simulink model "controller13_AIS"  (R2020b)
settings: Solver=FixedStepDiscrete  StartTime=0.0  StopTime=inf  RelTol=1e-3
values from neighbouring files (symbols this model uses):
  ctr = make_controller()    [setup_controller_with_functions.m]
  mdl = make_model(flight_time)    [setup_controller_with_functions.m]
  ukf_P0_flat = UKF.flatten_matrix(ukf_sys.P0)    [controller_setup_ukf.m]
  ukf_prediction_time = 0.015    [controller_setup_ukf.m]
  ukf_s0 = ukf_sys.s0    [controller_setup_ukf.m]
  ukf_sys = UKF.initialize_ukf_sys(rbt, mdl, ukf_params)    [controller_setup_ukf.m]
  ukf_use_prediction = 1    [controller_setup_ukf.m]
undefined symbols (not defined in the file or in its folder): ctr1, ctr2, DiscIntNeverNeededParam, flt, IO397, rbt1, rbt2, rsim1, rsim2, som, traj2
libraries: simulink x63, slrealtimeloglib x21, slrealtimetgmanagement x8, slrealtimeseriallib x5, speedgoatlib_fpga_analog_io x4, slrealtimeutilitieslib x3, dspfdesign x2, speedgoatlib_fpga x2, slrealtimeiplib x2, speedgoatlib_fpga_dio x1
(part 2 of 5)

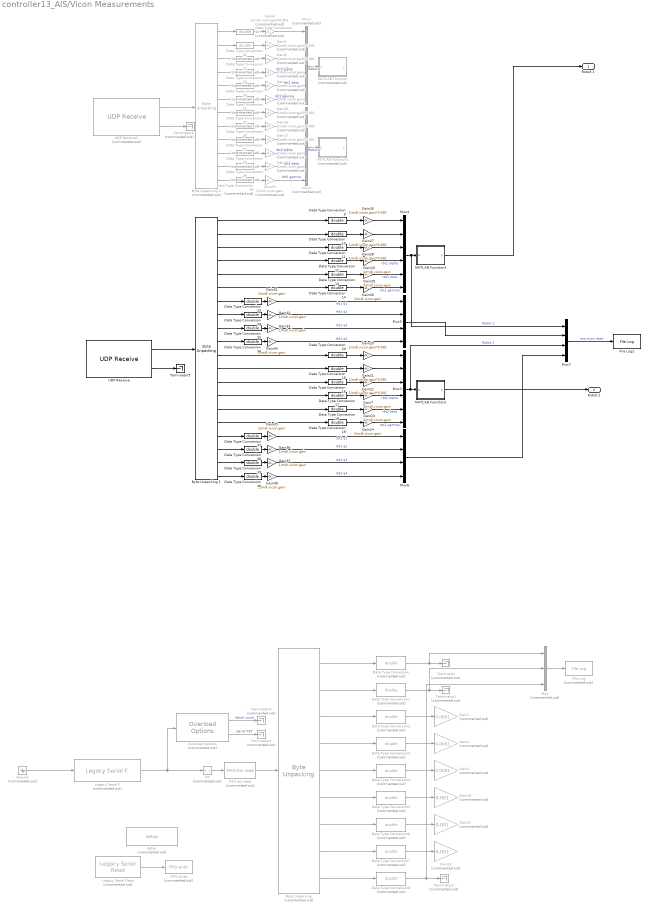
== system controller13_AIS/Vicon Measurements ==
  "Byte Unpacking " : slrealtimeutilitieslib/Byte Unpacking  Commented=on  MaskUnpackedDataTypes={'uint8','int16','int16','int16','int16','int16','int16','int16','uint8'}  MaskUnpackedDataSizes={[1] [1] [1] [1] [1] [1] [1] [1] [1]}  MaskAlignment=1
      settings: SourceProductBaseCode=XP
  Byte Unpacking 1 : slrealtimeutilitieslib/Byte Unpacking  MaskUnpackedDataTypes={'int32','int32','int32','int32','int32','int32','int32','int32','int32','int32','int32','int32','int32','int32','int32','int32','int32','int32','int32','int32'}  MaskUnpackedDataSizes={[1] [1] [1] [1] [1] [1] [1] [1] [1] [1] [1] [1] [1] [1] [1] [1] [1] [1] [1] [1]}  MaskAlignment=1
      settings: SourceProductBaseCode=XP
  Byte Unpacking 2 : slrealtimeutilitieslib/Byte Unpacking  Commented=on  MaskUnpackedDataTypes={'int32','int32','int32','int32','int32','int32','int32','int32','int32','int32','int32','int32'}  MaskUnpackedDataSizes={[1] [1] [1] [1] [1] [1] [1] [1] [1] [1] [1] [1]}  MaskAlignment=1
      settings: SourceProductBaseCode=XP
  Data Type Conversion{,1..8,21..32} (21 alike) : DataTypeConversion  Commented=on  OutDataTypeStr=double
  Data Type Conversion{9..20,33..40} (20 alike) : DataTypeConversion  OutDataTypeStr=double
  FIFO bin read : slrealtimeseriallib/FIFO bin read  Commented=on  header=[128,127,127]  lengths=[15]  hold=Hold last output if no new data  enable=off  maxsize=15  outputtype=8 bit uint null terminated  sampletime=mdl.T
      settings: SourceProductBaseCode=XP
  FIFO write : slrealtimeseriallib/FIFO write  Commented=on  size=1024  inputtype=count+16 bit uint  present=off  sampletime=-1
      settings: SourceProductBaseCode=XP
  File Log : slrealtimeloglib/File Log  Commented=on  decimation=1
      settings: SourceProductBaseCode=XP
  File Log1 : slrealtimeloglib/File Log  decimation=1
      settings: SourceProductBaseCode=XP
  Gain1 : Gain  Commented=on  Gain=0.0001
  Gain10 : Gain  Commented=on  Gain=0.001
  Gain11 : Gain  Commented=on  Gain=0.001
  Gain12 : Gain  Commented=on  Gain=0.001
  Gain{8..9,13..14,18..19} (6 alike) : Gain  Commented=on  Gain=1/mdl.vicon.gain
  Gain{4..6,15..17} (6 alike) : Gain  Commented=on  Gain=1/mdl.vicon.gain*0.001
  Gain2 : Gain  Commented=on  Gain=0.0001
  Gain{20..22,26..28} (6 alike) : Gain  Gain=1/mdl.vicon.gain*0.001
  Gain{7,23..25,29..38} (14 alike) : Gain  Gain=1/mdl.vicon.gain
  Gain3 : Gain  Commented=on  Gain=0.0001
  Ground : Ground  Commented=on
  Legacy Serial F : slrealtimeseriallib/Mainboard/Legacy Serial F  Commented=on  port=Legacy Serial Port 1  baud=115200  width=8  nstop=1  parity=None  ctsmode=on  idtype=8 bit uint null terminated  sampletime=0.0005
      settings: SourceProductBaseCode=XP
  Legacy Serial Read : slrealtimeseriallib/Mainboard/Legacy Serial Read  Commented=on  port=Legacy Serial Port 1  count=51  dtype=count+16 bit uint  sampletime=mdl.T
      settings: SourceProductBaseCode=XP
  MATLAB Function : MATLAB Function  Commented=on  TreatAsAtomicUnit=on  SystemSampleTime=mdl.T
  MATLAB Function1 : MATLAB Function  Commented=on  TreatAsAtomicUnit=on  SystemSampleTime=mdl.T
  MATLAB Function2 : MATLAB Function  TreatAsAtomicUnit=on  SystemSampleTime=mdl.T
  MATLAB Function3 : MATLAB Function  TreatAsAtomicUnit=on  SystemSampleTime=mdl.T
  Mux : Mux  Commented=on  Inputs=3
  Mux1 : Mux  Commented=on  Inputs=6
  Mux2 : Mux  Commented=on  Inputs=6
  Mux3 : Mux  Inputs=6
  Mux4 : Mux  Inputs=6
  Mux5 : Mux
  Mux6 : Mux
  Mux7 : Mux
  Overload Options : slrealtimetgmanagement/Overload Options  Commented=on  startupDur=10  startupDurSrc=Tunable Parameter  maxOverload=10  maxOverloadSrc=Tunable Parameter  TETFlag=on
      settings: SourceProductBaseCode=XP
  RT : RateTransition  Commented=on  Integrity=off  OutPortSampleTime=mdl.T
  Setup : slrealtimeseriallib/Mainboard/Setup  Commented=on  port=Legacy Serial Port 1  baud=115200  width=8  nstop=1  parity=None  ctsmode=on
      settings: SourceProductBaseCode=XP
  Terminator{,1..4,6} (6 alike) : Terminator  Commented=on
  Terminator5 : Terminator
  UDP Receive : slrealtimeiplib/UDP Receive  useHostTargetConn=off  ipAddress=192.168.8.11  localPort=1024  rcvWidth=80  rcvFmAny=on  fmAddress=192.168.7.11  rcvMulticast=off  multicastAddress={}  sampleTime=1/2500
      settings: SourceProductBaseCode=XP
  UDP Receive1 : slrealtimeiplib/UDP Receive  Commented=on  useHostTargetConn=off  ipAddress=192.168.8.11  localPort=1024  rcvWidth=48  rcvFmAny=on  fmAddress=192.168.7.11  rcvMulticast=off  multicastAddress={}  sampleTime=1/2500
      settings: SourceProductBaseCode=XP
  Robot 1 : Outport
  Robot 2 : Outport  Port=2
  wires:
  "Byte Unpacking "/3 -> Data Type Conversion2/1
  Data Type Conversion2/1 -> Gain1/1
  "Byte Unpacking "/9 -> Data Type Conversion8/1
  "Byte Unpacking "/4 -> Data Type Conversion3/1
  Data Type Conversion6/1 -> Gain11/1
  Data Type Conversion4/1 -> Gain3/1
  "Byte Unpacking "/2 -> Data Type Conversion1/1
  Data Type Conversion5/1 -> Gain10/1
  Data Type Conversion7/1 -> Gain12/1
  "Byte Unpacking "/6 -> Data Type Conversion5/1
  "Byte Unpacking "/8 -> Data Type Conversion7/1
  Data Type Conversion3/1 -> Gain2/1
  "Byte Unpacking "/5 -> Data Type Conversion4/1
  "Byte Unpacking "/7 -> Data Type Conversion6/1
  "Byte Unpacking "/1 -> Data Type Conversion/1
  Legacy Serial Read/1 -> FIFO write/1
  FIFO bin read/1 -> "Byte Unpacking "/1
  Ground/1 -> Legacy Serial F/1
  Legacy Serial F/1 -> Overload Options/1, RT/1
  RT/1 -> FIFO bin read/1
  Data Type Conversion/1 -> Mux/1, Terminator/1
  Data Type Conversion1/1 -> Mux/2, Terminator1/1
  Data Type Conversion8/1 -> Mux/3, Terminator2/1
  Mux/1 -> File Log/1
  Overload Options/1 -> Terminator4/1  "Serial count"
  Overload Options/2 -> Terminator3/1  "Serial TET"
  UDP Receive/2 -> Terminator5/1
  UDP Receive/1 -> Byte Unpacking 1/1
  Byte Unpacking 1/1 -> Data Type Conversion9/1
  Byte Unpacking 1/2 -> Data Type Conversion10/1
  Byte Unpacking 1/3 -> Data Type Conversion11/1
  Byte Unpacking 1/4 -> Data Type Conversion12/1
  Byte Unpacking 1/5 -> Data Type Conversion13/1
  Byte Unpacking 1/6 -> Data Type Conversion14/1
  Gain4/1 -> Mux1/1
  Gain5/1 -> Mux1/2
  Gain6/1 -> Mux1/3
  Gain13/1 -> Mux1/4  "rbt1 alpha"
  Gain8/1 -> Mux1/5  "rbt1 beta"
  Gain9/1 -> Mux1/6  "rbt1 gamma"
  Gain15/1 -> Mux2/1
  Gain16/1 -> Mux2/2
  Gain17/1 -> Mux2/3
  Gain14/1 -> Mux2/4  "rbt2 alpha"
  Gain18/1 -> Mux2/5  "rbt2 beta"
  Gain19/1 -> Mux2/6  "rbt2 gamma"
  Mux1/1 -> MATLAB Function/1(u)  "Robot 1"
  Mux2/1 -> MATLAB Function1/1(u)  "Robot 2"
  Byte Unpacking 2/12 -> Data Type Conversion30/1
  Byte Unpacking 2/9 -> Data Type Conversion27/1
  Byte Unpacking 2/7 -> Data Type Conversion31/1
  Byte Unpacking 2/3 -> Data Type Conversion22/1
  Byte Unpacking 2/6 -> Data Type Conversion25/1
  Byte Unpacking 2/4 -> Data Type Conversion23/1
  Byte Unpacking 2/10 -> Data Type Conversion28/1
  UDP Receive1/2 -> Terminator6/1
  Byte Unpacking 2/2 -> Data Type Conversion21/1
  Byte Unpacking 2/8 -> Data Type Conversion26/1
  UDP Receive1/1 -> Byte Unpacking 2/1
  Byte Unpacking 2/1 -> Data Type Conversion32/1
  Byte Unpacking 2/11 -> Data Type Conversion29/1
  Byte Unpacking 2/5 -> Data Type Conversion24/1
  Byte Unpacking 1/11 -> Data Type Conversion20/1
  Byte Unpacking 1/12 -> Data Type Conversion15/1
  Byte Unpacking 1/13 -> Data Type Conversion16/1
  Byte Unpacking 1/14 -> Data Type Conversion17/1
  Byte Unpacking 1/15 -> Data Type Conversion18/1
  Byte Unpacking 1/16 -> Data Type Conversion19/1
  Data Type Conversion33/1 -> Gain31/1
  Gain31/1 -> Mux5/1  "rbt1 q1"
  Byte Unpacking 1/7 -> Data Type Conversion33/1
  Data Type Conversion34/1 -> Gain32/1
  Gain32/1 -> Mux5/2  "rbt1 q2"
  Byte Unpacking 1/8 -> Data Type Conversion34/1
  Data Type Conversion35/1 -> Gain33/1
  Data Type Conversion36/1 -> Gain34/1
  Byte Unpacking 1/9 -> Data Type Conversion35/1
  Byte Unpacking 1/10 -> Data Type Conversion36/1
  Gain33/1 -> Mux5/3  "rbt1 q3"
  Gain34/1 -> Mux5/4  "rbt1 q4"
  Gain38/1 -> Mux6/4  "rbt2 q4"
  Gain37/1 -> Mux6/3  "rbt2 q3"
  Data Type Conversion37/1 -> Gain35/1
  Gain35/1 -> Mux6/1  "rbt2 q1"
  Data Type Conversion40/1 -> Gain38/1
  Data Type Conversion38/1 -> Gain36/1
  Gain36/1 -> Mux6/2  "rbt2 q2"
  Data Type Conversion39/1 -> Gain37/1
  Byte Unpacking 1/17 -> Data Type Conversion37/1
  Byte Unpacking 1/18 -> Data Type Conversion38/1
  Byte Unpacking 1/19 -> Data Type Conversion39/1
  Byte Unpacking 1/20 -> Data Type Conversion40/1
  Data Type Conversion32/1 -> Gain4/1
  Data Type Conversion21/1 -> Gain5/1
  Data Type Conversion23/1 -> Gain13/1
  Data Type Conversion22/1 -> Gain6/1
  Data Type Conversion24/1 -> Gain8/1
  Data Type Conversion25/1 -> Gain9/1
  Data Type Conversion31/1 -> Gain15/1
  Data Type Conversion26/1 -> Gain16/1
  Data Type Conversion27/1 -> Gain17/1
  Data Type Conversion28/1 -> Gain14/1
  Data Type Conversion29/1 -> Gain18/1
  Data Type Conversion30/1 -> Gain19/1
  Gain23/1 -> Mux3/5  "rbt2 beta"
  Gain7/1 -> Mux3/4  "rbt2 alpha"
  Gain22/1 -> Mux3/3
  Mux3/1 -> Mux7/3, MATLAB Function2/1(u)  "Robot 2"
  Gain24/1 -> Mux3/6  "rbt2 gamma"
  Gain20/1 -> Mux3/1
  Gain21/1 -> Mux3/2
  Data Type Conversion20/1 -> Gain20/1
  Data Type Conversion15/1 -> Gain21/1
  Data Type Conversion16/1 -> Gain22/1
  Data Type Conversion17/1 -> Gain7/1
  Data Type Conversion18/1 -> Gain23/1
  Data Type Conversion19/1 -> Gain24/1
  Gain26/1 -> Mux4/1
  Gain27/1 -> Mux4/2
  Gain30/1 -> Mux4/6  "rbt1 gamma"
  Mux4/1 -> Mux7/1, MATLAB Function3/1(u)  "Robot 1"
  Gain28/1 -> Mux4/3
  Gain29/1 -> Mux4/5  "rbt1 beta"
  Gain25/1 -> Mux4/4  "rbt1 alpha"
  Data Type Conversion9/1 -> Gain26/1
  Data Type Conversion10/1 -> Gain27/1
  Data Type Conversion11/1 -> Gain28/1
  Data Type Conversion12/1 -> Gain25/1
  Data Type Conversion13/1 -> Gain29/1
  Data Type Conversion14/1 -> Gain30/1
  MATLAB Function3/1(y) -> Robot 1/1
  MATLAB Function2/1(y) -> Robot 2/1
  Mux7/1 -> File Log1/1  "raw vicon data"
  Mux5/1 -> Mux7/2
  Mux6/1 -> Mux7/4

== system controller13_AIS/closed loop en 1 ==
  x tor : Inport
  y tor : Inport  Port=2
  z tor : Inport  Port=3
  thurst : Inport  Port=4
  enable : Constant  Value=ctr1.en
  enable{1..4} (4 alike) : Product  Inputs=**
  safety1 : Subsystem
  safety2 : Subsystem
  safety3 : Subsystem
  safety4 : Subsystem
  tor x : Outport
  tor y : Outport  Port=2
  tor z : Outport  Port=3
  Force : Outport  Port=4
  wires:
  enable/1 -> enable2/1, enable3/1, enable4/1, enable1/1
  z tor/1 -> enable3/2
  y tor/1 -> enable2/2
  x tor/1 -> enable1/2
  thurst/1 -> enable4/2
  enable1/1 -> safety1/1(In1)
  enable2/1 -> safety2/1(In1)
  enable3/1 -> safety3/1(In1)
  enable4/1 -> safety4/1(In1)
  safety1/1(Out1) -> tor x/1
  safety2/1(Out1) -> tor y/1
  safety3/1(Out1) -> tor z/1
  safety4/1(Out1) -> Force/1

== system controller13_AIS/closed loop en 2 ==
  x tor : Inport
  y tor : Inport  Port=2
  z tor : Inport  Port=3
  thurst : Inport  Port=4
  enable : Constant  Value=ctr2.en
  enable{1..4} (4 alike) : Product  Inputs=**
  safety1 : Subsystem
  safety2 : Subsystem
  safety3 : Subsystem
  safety4 : Subsystem
  tor x : Outport
  tor y : Outport  Port=2
  tor z : Outport  Port=3
  Force : Outport  Port=4
  wires:
  enable/1 -> enable2/1, enable3/1, enable4/1, enable1/1
  z tor/1 -> enable3/2
  y tor/1 -> enable2/2
  x tor/1 -> enable1/2
  thurst/1 -> enable4/2
  enable1/1 -> safety1/1(In1)
  enable2/1 -> safety2/1(In1)
  enable3/1 -> safety3/1(In1)
  enable4/1 -> safety4/1(In1)
  safety1/1(Out1) -> tor x/1
  safety2/1(Out1) -> tor y/1
  safety3/1(Out1) -> tor z/1
  safety4/1(Out1) -> Force/1

== system controller13_AIS/counter 1 ==
  running time : Inport
  Add : Sum  Inputs=+-
  Add1 : Sum
  Compare To Zero : simulink/Logic and Bit Operations/Compare To Zero  relop=<  OutDataTypeStr=uint8  ZeroCross=off
  Product2 : Product  RndMeth=Zero
  Relational Operator : RelationalOperator  Operator=>  OutDataTypeStr=boolean  RndMeth=Simplest
  SaturatingRamp : DiscreteIntegrator  gainval=1  SampleTime=-1  UpperSaturationLimit=1  LowerSaturationLimit=0  ICPrevOutput=DiscIntNeverNeededParam  ICPrevScaledInput=DiscIntNeverNeededParam
  Stop Simulation : Stop
  constant : Constant
  start delay compare : simulink/Logic and Bit Operations/Compare To Constant  relop=>  const=mdl.i_delay  OutDataTypeStr=uint8
  enable : Outport
  wires:
  SaturatingRamp/1 -> Relational Operator/1, Add/1, start delay compare/1
  running time/1 -> Add1/2, Add/2
  Add/1 -> Compare To Zero/1
  start delay compare/1 -> Product2/1
  Compare To Zero/1 -> Product2/2
  Product2/1 -> enable/1
  constant/1 -> Add1/1, SaturatingRamp/1
  Relational Operator/1 -> Stop Simulation/1
  Add1/1 -> Relational Operator/2

== system controller13_AIS/counter 2 ==
  running time : Inport
  Add : Sum  Inputs=+-
  Add1 : Sum
  Compare To Zero : simulink/Logic and Bit Operations/Compare To Zero  relop=<  OutDataTypeStr=uint8  ZeroCross=off
  Product2 : Product  RndMeth=Zero
  Relational Operator : RelationalOperator  Operator=>  OutDataTypeStr=boolean  RndMeth=Simplest
  SaturatingRamp : DiscreteIntegrator  gainval=1  SampleTime=-1  UpperSaturationLimit=1  LowerSaturationLimit=0  ICPrevOutput=DiscIntNeverNeededParam  ICPrevScaledInput=DiscIntNeverNeededParam
  Stop Simulation : Stop
  constant : Constant
  start delay compare : simulink/Logic and Bit Operations/Compare To Constant  relop=>  const=mdl.i_delay  OutDataTypeStr=uint8
  enable : Outport
  wires:
  SaturatingRamp/1 -> Relational Operator/1, Add/1, start delay compare/1
  running time/1 -> Add1/2, Add/2
  Add/1 -> Compare To Zero/1
  start delay compare/1 -> Product2/1
  Compare To Zero/1 -> Product2/2
  Product2/1 -> enable/1
  constant/1 -> Add1/1, SaturatingRamp/1
  Relational Operator/1 -> Stop Simulation/1
  Add1/1 -> Relational Operator/2

== system controller13_AIS/disturbance 1 ==
  Constant : Constant  Value=rsim1.dist.pos.en
  Constant1 : Constant  Value=[0;0;0;]
  Constant2 : Constant  Value=rsim1.dist.rot.en
  Constant3 : Constant  Value=[0;0;0;]
  Mux1 : Mux  Inputs=3
  Mux2 : Mux  Inputs=3
  Mux3 : Mux  Inputs=2
  Random Number : RandomNumber  Mean=rsim1.dist.x.mean  Variance=rsim1.dist.x.var  Seed=rsim1.dist.x.seed
  Random Number1 : RandomNumber  Mean=rsim1.dist.y.mean  Variance=rsim1.dist.y.var  Seed=rsim1.dist.y.seed
  Random Number2 : RandomNumber  Mean=rsim1.dist.z.mean  Variance=rsim1.dist.z.var  Seed=rsim1.dist.z.seed
  Random Number3 : RandomNumber  Mean=rsim1.dist.wx.mean  Variance=rsim1.dist.wx.var  Seed=rsim1.dist.wx.seed
  Random Number4 : RandomNumber  Mean=rsim1.dist.wy.mean  Variance=rsim1.dist.wy.var  Seed=rsim1.dist.wy.seed
  Random Number5 : RandomNumber  Mean=rsim1.dist.wz.mean  Variance=rsim1.dist.wz.var  Seed=rsim1.dist.wz.seed
  Switch : Switch  Threshold=1
  Switch1 : Switch  Threshold=1
  disturbance : Outport  VectorParamsAs1DForOutWhenUnconnected=off
  wires:
  Random Number/1 -> Mux1/1
  Random Number2/1 -> Mux1/3
  Mux1/1 -> Switch/1
  Random Number1/1 -> Mux1/2
  Switch/1 -> Mux3/1
  Constant/1 -> Switch/2
  Constant1/1 -> Switch/3
  Mux2/1 -> Switch1/1
  Random Number5/1 -> Mux2/3
  Constant3/1 -> Switch1/3
  Constant2/1 -> Switch1/2
  Random Number4/1 -> Mux2/2
  Random Number3/1 -> Mux2/1
  Switch1/1 -> Mux3/2
  Mux3/1 -> disturbance/1

== system controller13_AIS/disturbance 2 ==
  Constant : Constant  Value=rsim2.dist.pos.en
  Constant1 : Constant  Value=[0;0;0;]
  Constant2 : Constant  Value=rsim2.dist.rot.en
  Constant3 : Constant  Value=[0;0;0;]
  Mux1 : Mux  Inputs=3
  Mux2 : Mux  Inputs=3
  Mux3 : Mux  Inputs=2
  Random Number : RandomNumber  Mean=rsim2.dist.x.mean  Variance=rsim2.dist.x.var  Seed=rsim2.dist.x.seed
  Random Number1 : RandomNumber  Mean=rsim2.dist.y.mean  Variance=rsim2.dist.y.var  Seed=rsim2.dist.y.seed
  Random Number2 : RandomNumber  Mean=rsim2.dist.z.mean  Variance=rsim2.dist.z.var  Seed=rsim2.dist.z.seed
  Random Number3 : RandomNumber  Mean=rsim2.dist.wx.mean  Variance=rsim2.dist.wx.var  Seed=rsim2.dist.wx.seed
  Random Number4 : RandomNumber  Mean=rsim2.dist.wy.mean  Variance=rsim2.dist.wy.var  Seed=rsim2.dist.wy.seed
  Random Number5 : RandomNumber  Mean=rsim2.dist.wz.mean  Variance=rsim2.dist.wz.var  Seed=rsim2.dist.wz.seed
  Switch : Switch  Threshold=1
  Switch1 : Switch  Threshold=1
  disturbance : Outport  VectorParamsAs1DForOutWhenUnconnected=off
  wires:
  Random Number/1 -> Mux1/1
  Random Number2/1 -> Mux1/3
  Mux1/1 -> Switch/1
  Random Number1/1 -> Mux1/2
  Switch/1 -> Mux3/1
  Constant/1 -> Switch/2
  Constant1/1 -> Switch/3
  Mux2/1 -> Switch1/1
  Random Number5/1 -> Mux2/3
  Constant3/1 -> Switch1/3
  Constant2/1 -> Switch1/2
  Random Number4/1 -> Mux2/2
  Random Number3/1 -> Mux2/1
  Switch1/1 -> Mux3/2
  Mux3/1 -> disturbance/1

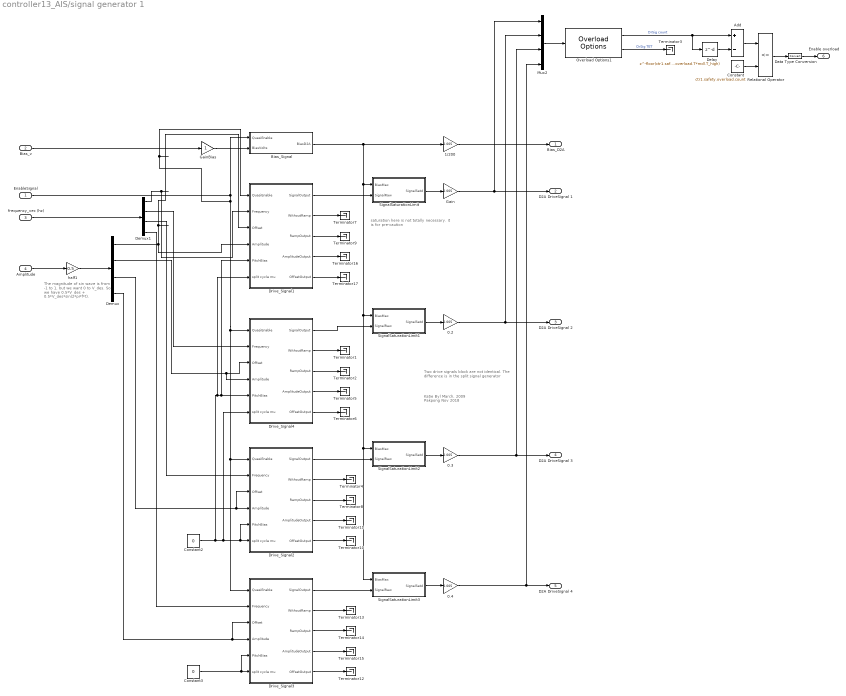
== system controller13_AIS/signal generator 1 ==
  note: The magnitude of sin wave is from -1 to 1, but we want 0 to V_des. So we have 0.5*V_des + 0.5*V_des*sin(2*pi*f*t).
  note: Katie Byl
      | March, 2009
      |
      | Pakpong
      | Nov 2018
  note: Two drive signals block are not identical.
      | The difference is in the split signal generator
  note: saturation here is not totally necessary.
      | it is for pre-caution
  EnableSignal : Inport
  Bias_v : Inport  Port=2
  frequency_vec (hz) : Inport  Port=3
  Amplitude : Inport  Port=4
  0.2 : Gain  Gain=0.005
  0.3 : Gain  Gain=0.005
  0.4 : Gain  Gain=0.005
  1/200 : Gain  Gain=0.005
  Add : Sum  Inputs=+-
  Bias_Signal : Subsystem
  Constant : Constant  Value=ctr1.safety.overload.count
  Constant2 : Constant  Value=0
  Constant3 : Constant  Value=0
  Data Type Conversion : DataTypeConversion
  Delay : Delay  DelayLength=floor(ctr1.safety.overload.T*mdl.T_high)  InitialCondition=0
  Demux : Demux
  Demux1 : Demux
  Drive_Signal1 : Subsystem
  Drive_Signal2 : Subsystem
  Drive_Signal3 : Subsystem
  Drive_Signal4 : Subsystem
  Gain : Gain  Gain=0.005
  GainBias : Gain
  Mux2 : Mux
  Overload Options1 : slrealtimetgmanagement/Overload Options  startupDur=10  startupDurSrc=Tunable Parameter  maxOverload=1000  maxOverloadSrc=Tunable Parameter  TETFlag=on
      settings: SourceProductBaseCode=XP
  Relational Operator : RelationalOperator  Operator=<=  OutDataTypeStr=boolean  RndMeth=Simplest
  SignalSaturationLimit : Subsystem
  SignalSaturationLimit1 : Subsystem
  SignalSaturationLimit2 : Subsystem
  SignalSaturationLimit3 : Subsystem
  Terminator{1..17} (17 alike) : Terminator
  half1 : Gain  Gain=0.5
  Bias_D2A : Outport
  D2A DriveSignal 1 : Outport  Port=2
  D2A DriveSignal 2 : Outport  Port=3
  D2A DriveSignal 3 : Outport  Port=4
  D2A DriveSignal 4 : Outport  Port=5
  Enable overload : Outport  Port=6
  wires:
  Bias_Signal/1(BiasD2A) -> SignalSaturationLimit3/1(BiasMax), SignalSaturationLimit2/1(BiasMax), SignalSaturationLimit1/1(BiasMax), SignalSaturationLimit/1(BiasMax), 1/200/1
  Bias_v/1 -> GainBias/1
  EnableSignal/1 -> Drive_Signal1/1(QuasiEnable), Drive_Signal3/1(QuasiEnable), Drive_Signal2/1(QuasiEnable), Drive_Signal4/1(QuasiEnable), Bias_Signal/1(QuasiEnable)
  SignalSaturationLimit/1(SignalSatd) -> Gain/1
  GainBias/1 -> Bias_Signal/2(BiasVolts)
  SignalSaturationLimit1/1(SignalSatd) -> 0.2/1
  Amplitude/1 -> half1/1
  1/200/1 -> Bias_D2A/1
  Gain/1 -> Mux2/1, D2A DriveSignal 1/1
  Drive_Signal3/4(AmplitudeOutput) -> Terminator15/1
  Drive_Signal3/2(WithoutRamp) -> Terminator13/1
  Drive_Signal3/3(RampOutput) -> Terminator14/1
  Drive_Signal3/5(OffsetOutput) -> Terminator12/1
  Drive_Signal2/3(RampOutput) -> Terminator8/1
  Drive_Signal2/4(AmplitudeOutput) -> Terminator11/1
  Drive_Signal3/1(SignalOutput) -> SignalSaturationLimit3/2(SignalRaw)
  Drive_Signal2/5(OffsetOutput) -> Terminator10/1
  Drive_Signal2/2(WithoutRamp) -> Terminator4/1
  Demux/2 -> Drive_Signal4/4(Amplitude), Drive_Signal4/3(Offset)
  Demux/3 -> Drive_Signal2/4(Amplitude), Drive_Signal2/3(Offset)
  Demux/4 -> Drive_Signal3/4(Amplitude), Drive_Signal3/3(Offset)
  Constant2/1 -> Drive_Signal1/6(split cycle mu), Drive_Signal1/5(PitchBias), Drive_Signal4/5(PitchBias), Drive_Signal4/6(split cycle mu), Drive_Signal2/5(PitchBias), Drive_Signal2/6(split cycle mu)
  Constant3/1 -> Drive_Signal3/5(PitchBias), Drive_Signal3/6(split cycle mu)
  0.3/1 -> D2A DriveSignal 3/1, Mux2/3
  SignalSaturationLimit2/1(SignalSatd) -> 0.3/1
  0.4/1 -> D2A DriveSignal 4/1, Mux2/4
  SignalSaturationLimit3/1(SignalSatd) -> 0.4/1
  Drive_Signal2/1(SignalOutput) -> SignalSaturationLimit2/2(SignalRaw)
  half1/1 -> Demux/1
  frequency_vec (hz)/1 -> Demux1/1
  Demux1/1 -> Drive_Signal1/2(Frequency)
  Demux1/2 -> Drive_Signal4/2(Frequency)
  Demux1/3 -> Drive_Signal2/2(Frequency)
  Demux1/4 -> Drive_Signal3/2(Frequency)
  0.2/1 -> Mux2/2, D2A DriveSignal 2/1
  Overload Options1/1 -> Delay/1, Add/1  "DrSig count"
  Overload Options1/2 -> Terminator3/1  "DrSig TET"
  Mux2/1 -> Overload Options1/1
  Delay/1 -> Add/2
  Add/1 -> Relational Operator/1
  Constant/1 -> Relational Operator/2
  Relational Operator/1 -> Data Type Conversion/1
  Data Type Conversion/1 -> Enable overload/1
  Drive_Signal4/1(SignalOutput) -> SignalSaturationLimit1/2(SignalRaw)
  Drive_Signal4/2(WithoutRamp) -> Terminator1/1
  Drive_Signal4/3(RampOutput) -> Terminator2/1
  Drive_Signal4/4(AmplitudeOutput) -> Terminator5/1
  Drive_Signal4/5(OffsetOutput) -> Terminator6/1
  Drive_Signal1/4(AmplitudeOutput) -> Terminator16/1
  Drive_Signal1/1(SignalOutput) -> SignalSaturationLimit/2(SignalRaw)
  Drive_Signal1/2(WithoutRamp) -> Terminator7/1
  Drive_Signal1/5(OffsetOutput) -> Terminator17/1
  Drive_Signal1/3(RampOutput) -> Terminator9/1
  Demux/1 -> Drive_Signal1/3(Offset), Drive_Signal1/4(Amplitude)

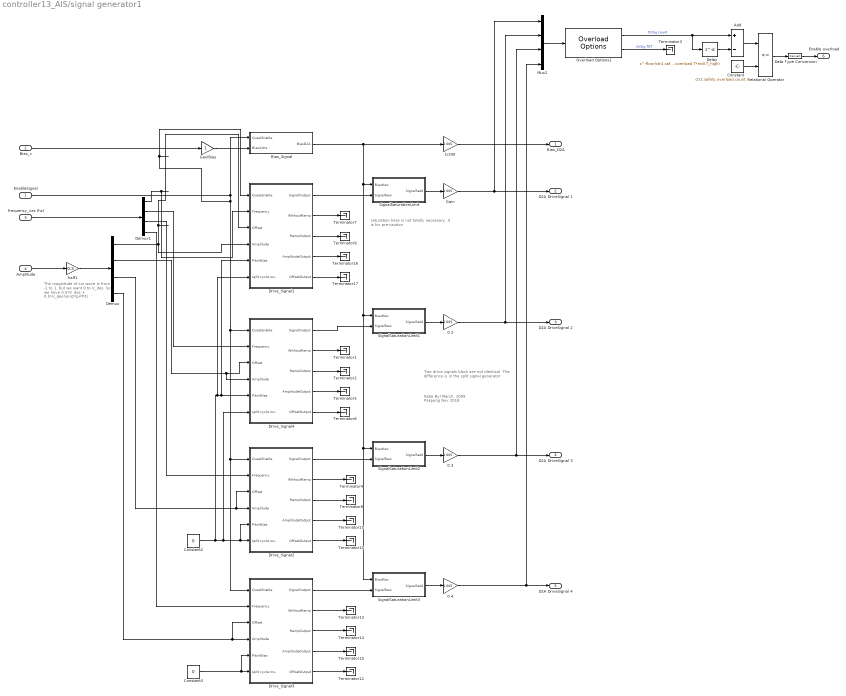
== system controller13_AIS/signal generator1 ==
  note: The magnitude of sin wave is from -1 to 1, but we want 0 to V_des. So we have 0.5*V_des + 0.5*V_des*sin(2*pi*f*t).
  note: Katie Byl
      | March, 2009
      |
      | Pakpong
      | Nov 2018
  note: Two drive signals block are not identical.
      | The difference is in the split signal generator
  note: saturation here is not totally necessary.
      | it is for pre-caution
  EnableSignal : Inport
  Bias_v : Inport  Port=2
  frequency_vec (hz) : Inport  Port=3
  Amplitude : Inport  Port=4
  0.2 : Gain  Gain=0.005
  0.3 : Gain  Gain=0.005
  0.4 : Gain  Gain=0.005
  1/200 : Gain  Gain=0.005
  Add : Sum  Inputs=+-
  Bias_Signal : Subsystem
  Constant : Constant  Value=ctr2.safety.overload.count
  Constant2 : Constant  Value=0
  Constant3 : Constant  Value=0
  Data Type Conversion : DataTypeConversion
  Delay : Delay  DelayLength=floor(ctr2.safety.overload.T*mdl.T_high)  InitialCondition=0
  Demux : Demux
  Demux1 : Demux
  Drive_Signal1 : Subsystem
  Drive_Signal2 : Subsystem
  Drive_Signal3 : Subsystem
  Drive_Signal4 : Subsystem
  Gain : Gain  Gain=0.005
  GainBias : Gain
  Mux2 : Mux
  Overload Options1 : slrealtimetgmanagement/Overload Options  startupDur=10  startupDurSrc=Tunable Parameter  maxOverload=1000  maxOverloadSrc=Tunable Parameter  TETFlag=on
      settings: SourceProductBaseCode=XP
  Relational Operator : RelationalOperator  Operator=<=  OutDataTypeStr=boolean  RndMeth=Simplest
  SignalSaturationLimit : Subsystem
  SignalSaturationLimit1 : Subsystem
  SignalSaturationLimit2 : Subsystem
  SignalSaturationLimit3 : Subsystem
  Terminator{1..17} (17 alike) : Terminator
  half1 : Gain  Gain=0.5
  Bias_D2A : Outport
  D2A DriveSignal 1 : Outport  Port=2
  D2A DriveSignal 2 : Outport  Port=3
  D2A DriveSignal 3 : Outport  Port=4
  D2A DriveSignal 4 : Outport  Port=5
  Enable overload : Outport  Port=6
  wires:
  Bias_Signal/1(BiasD2A) -> SignalSaturationLimit3/1(BiasMax), SignalSaturationLimit2/1(BiasMax), SignalSaturationLimit1/1(BiasMax), SignalSaturationLimit/1(BiasMax), 1/200/1
  Bias_v/1 -> GainBias/1
  EnableSignal/1 -> Drive_Signal1/1(QuasiEnable), Drive_Signal3/1(QuasiEnable), Drive_Signal2/1(QuasiEnable), Drive_Signal4/1(QuasiEnable), Bias_Signal/1(QuasiEnable)
  SignalSaturationLimit/1(SignalSatd) -> Gain/1
  GainBias/1 -> Bias_Signal/2(BiasVolts)
  SignalSaturationLimit1/1(SignalSatd) -> 0.2/1
  Amplitude/1 -> half1/1
  1/200/1 -> Bias_D2A/1
  Gain/1 -> Mux2/1, D2A DriveSignal 1/1
  Drive_Signal3/4(AmplitudeOutput) -> Terminator15/1
  Drive_Signal3/2(WithoutRamp) -> Terminator13/1
  Drive_Signal3/3(RampOutput) -> Terminator14/1
  Drive_Signal3/5(OffsetOutput) -> Terminator12/1
  Drive_Signal2/3(RampOutput) -> Terminator8/1
  Drive_Signal2/4(AmplitudeOutput) -> Terminator11/1
  Drive_Signal3/1(SignalOutput) -> SignalSaturationLimit3/2(SignalRaw)
  Drive_Signal2/5(OffsetOutput) -> Terminator10/1
  Drive_Signal2/2(WithoutRamp) -> Terminator4/1
  Demux/2 -> Drive_Signal4/4(Amplitude), Drive_Signal4/3(Offset)
  Demux/3 -> Drive_Signal2/4(Amplitude), Drive_Signal2/3(Offset)
  Demux/4 -> Drive_Signal3/4(Amplitude), Drive_Signal3/3(Offset)
  Constant2/1 -> Drive_Signal1/6(split cycle mu), Drive_Signal1/5(PitchBias), Drive_Signal4/5(PitchBias), Drive_Signal4/6(split cycle mu), Drive_Signal2/5(PitchBias), Drive_Signal2/6(split cycle mu)
  Constant3/1 -> Drive_Signal3/5(PitchBias), Drive_Signal3/6(split cycle mu)
  0.3/1 -> D2A DriveSignal 3/1, Mux2/3
  SignalSaturationLimit2/1(SignalSatd) -> 0.3/1
  0.4/1 -> D2A DriveSignal 4/1, Mux2/4
  SignalSaturationLimit3/1(SignalSatd) -> 0.4/1
  Drive_Signal2/1(SignalOutput) -> SignalSaturationLimit2/2(SignalRaw)
  half1/1 -> Demux/1
  frequency_vec (hz)/1 -> Demux1/1
  Demux1/1 -> Drive_Signal1/2(Frequency)
  Demux1/2 -> Drive_Signal4/2(Frequency)
  Demux1/3 -> Drive_Signal2/2(Frequency)
  Demux1/4 -> Drive_Signal3/2(Frequency)
  0.2/1 -> Mux2/2, D2A DriveSignal 2/1
  Overload Options1/1 -> Delay/1, Add/1  "DrSig count"
  Overload Options1/2 -> Terminator3/1  "DrSig TET"
  Mux2/1 -> Overload Options1/1
  Delay/1 -> Add/2
  Add/1 -> Relational Operator/1
  Constant/1 -> Relational Operator/2
  Relational Operator/1 -> Data Type Conversion/1
  Data Type Conversion/1 -> Enable overload/1
  Drive_Signal4/1(SignalOutput) -> SignalSaturationLimit1/2(SignalRaw)
  Drive_Signal4/2(WithoutRamp) -> Terminator1/1
  Drive_Signal4/3(RampOutput) -> Terminator2/1
  Drive_Signal4/4(AmplitudeOutput) -> Terminator5/1
  Drive_Signal4/5(OffsetOutput) -> Terminator6/1
  Drive_Signal1/4(AmplitudeOutput) -> Terminator16/1
  Drive_Signal1/1(SignalOutput) -> SignalSaturationLimit/2(SignalRaw)
  Drive_Signal1/2(WithoutRamp) -> Terminator7/1
  Drive_Signal1/5(OffsetOutput) -> Terminator17/1
  Drive_Signal1/3(RampOutput) -> Terminator9/1
  Demux/1 -> Drive_Signal1/3(Offset), Drive_Signal1/4(Amplitude)

== system controller13_AIS/smothing 1 ==
  amp : Inport
  Delay : Delay  DelayLength=1
  SaturatingRamp : DiscreteIntegrator  gainval=1  SampleTime=-1  UpperSaturationLimit=1  LowerSaturationLimit=0  ICPrevOutput=DiscIntNeverNeededParam  ICPrevScaledInput=DiscIntNeverNeededParam
  constant : Constant
  smoothing : MATLAB Function  TreatAsAtomicUnit=on
  control voltage : Outport
  wires:
  smoothing/1(out_amp) -> Delay/1, control voltage/1
  amp/1 -> smoothing/2(amp)
  Delay/1 -> smoothing/3(amp2)
  constant/1 -> SaturatingRamp/1
  SaturatingRamp/1 -> smoothing/1(time)

== system controller13_AIS/smothing 2 ==
  amp : Inport
  Delay : Delay  DelayLength=1
  SaturatingRamp : DiscreteIntegrator  gainval=1  SampleTime=-1  UpperSaturationLimit=1  LowerSaturationLimit=0  ICPrevOutput=DiscIntNeverNeededParam  ICPrevScaledInput=DiscIntNeverNeededParam
  constant : Constant
  smoothing : MATLAB Function  TreatAsAtomicUnit=on
  control voltage : Outport
  wires:
  smoothing/1(out_amp) -> Delay/1, control voltage/1
  amp/1 -> smoothing/2(amp)
  Delay/1 -> smoothing/3(amp2)
  constant/1 -> SaturatingRamp/1
  SaturatingRamp/1 -> smoothing/1(time)

== system controller13_AIS/z Amplifier Measurement ==
  Amplifier : slrealtimeloglib/File Log  decimation=1
      settings: SourceProductBaseCode=XP
  Constant : Constant
  IO397 Analog Input : speedgoatlib_fpga_analog_io/IO397 Analog Input  Commented=on  id=1  chan=[1:4]  range=+-10.24 V  trigger=Initiator  ts=mdl.T_high  pciSlot=[6,0]  board=IO397-50k
      settings: SourceProductName=Simulink Real-Time: Speedgoat Library
  IO397 Analog Input1 : speedgoatlib_fpga_analog_io/IO397 Analog Input  Commented=on  id=2  chan=[1:4]  range=+-10.24 V  trigger=Initiator  ts=mdl.T_high  pciSlot=[11,0]  board=IO397-50k
      settings: SourceProductName=Simulink Real-Time: Speedgoat Library
  Mux : Mux  Commented=on  Inputs=8
  Overload Options : slrealtimetgmanagement/Overload Options  Commented=on  startupDur=10  startupDurSrc=Tunable Parameter  maxOverload=1000  maxOverloadSrc=Tunable Parameter  TETFlag=on
      settings: SourceProductBaseCode=XP
  Terminator1 : Terminator  Commented=on
  Terminator2 : Terminator  Commented=on
  wires:
  IO397 Analog Input/4 -> Mux/4  "mdl1 s4"
  IO397 Analog Input/2 -> Mux/2  "mdl1 s2"
  IO397 Analog Input/1 -> Mux/1  "mdl1 s1"
  IO397 Analog Input/3 -> Mux/3  "mdl1 s3"
  IO397 Analog Input1/1 -> Mux/5
  IO397 Analog Input1/2 -> Mux/6
  IO397 Analog Input1/3 -> Mux/7
  IO397 Analog Input1/4 -> Mux/8
  Mux/1 -> Overload Options/1
  Overload Options/1 -> Terminator2/1  "Sensing count"
  Overload Options/2 -> Terminator1/1  "Sensing TET"
  Constant/1 -> Amplifier/1  "sensing"

== system controller13_AIS/Adaptive Controller 1/adaptive system ==
  att_e : Inport
  alt_e : Inport  Port=2
  Mux : Mux  Inputs=2
  Saturation1 : Saturate  UpperLimit=1  LowerLimit=-1
  Saturation3 : Saturate  UpperLimit=0.06  LowerLimit=-0.06
  Scope : Scope
  Unit Delay : UnitDelay  SampleTime=-1  HasFrameUpgradeWarning=on
  enable1 : Product  Inputs=**
  integral enable : Constant  Value=ctr1.integral.en
  integrator : Subsystem
  safety1 : Subsystem
  safety2 : Subsystem
  thrust offset : Constant  Value=flt.thrust_off
  torque offset : Constant  Value=[flt.torx_off;flt.tory_off;flt.torz_off]
  " tor_off" : Outport
  th_off : Outport  Port=2
  int_e : Outport  Port=3
  wires:
  torque offset/1 -> integrator/2(torque offset)
  thrust offset/1 -> integrator/3(thrust_offset)
  integrator/3(th_off) -> th_off/1
  integrator/1(int_e) -> Unit Delay/1
  integral enable/1 -> enable1/1
  Mux/1 -> integrator/1(e)
  Unit Delay/1 -> enable1/2
  integrator/2(" torq_off") -> Scope/1, " tor_off"/1
  att_e/1 -> safety1/1(In1)
  enable1/1 -> int_e/1
  alt_e/1 -> safety2/1(In1)
  Saturation1/1 -> Mux/1
  Saturation3/1 -> Mux/2
  safety1/1(Out1) -> Saturation1/1
  safety2/1(Out1) -> Saturation3/1

== system controller13_AIS/Adaptive Controller 1/attitude and thrust controller ==
  note: x_hat_pred
  r : Inport
  r_dot : Inport  Port=2
  r_dotdot : Inport  Port=3
  R : Inport  Port=4
  Omega : Inport  Port=5
  rd : Inport  Port=6
  rd_d : Inport  Port=7
  rd_dd : Inport  Port=8
  rd_ddd : Inport  Port=9
  rd_dddd : Inport  Port=10
  int_e : Inport  Port=11
  euler angle : Inport  Port=12
  Attitude Controleller : MATLAB Function  TreatAsAtomicUnit=on
  Delay : Delay  DelayLength=1  InitialCondition=ctr1.torque_obs.ext_torq_hat_init  SampleTime=mdl.T
  Delay1 : Delay  DelayLength=1  InitialCondition=ctr1.torque_obs.omega_hat_init  SampleTime=mdl.T
  External Torque Observer : MATLAB Function  TreatAsAtomicUnit=on
  Terminator2 : Terminator
  Thrust Controller : MATLAB Function  TreatAsAtomicUnit=on
  Yaw Controller : Subsystem
  rd1 : slrealtimeloglib/File Log  decimation=1
      settings: SourceProductBaseCode=XP
  time : Subsystem
  torque_x : Outport
  torque_y : Outport  Port=2
  torque_z : Outport  Port=3
  F : Outport  Port=4
  att_e : Outport  Port=5
  alt_e : Outport  Port=6
  wires:
  r/1 -> Thrust Controller/1(r), Attitude Controleller/1(r)
  Attitude Controleller/1(torque_x) -> External Torque Observer/2(torque_x), torque_x/1
  r_dot/1 -> Attitude Controleller/2(r_dot), Thrust Controller/2(r_dot)
  r_dotdot/1 -> Attitude Controleller/3(r_dotdot), Thrust Controller/3(r_dotdot)
  R/1 -> Attitude Controleller/4(R), Thrust Controller/4(R)
  Attitude Controleller/2(torque_y) -> External Torque Observer/3(torque_y), torque_y/1
  Omega/1 -> Attitude Controleller/5(Omega), External Torque Observer/1(omega), Thrust Controller/5(Omega)
  rd/1 -> Attitude Controleller/6(rd), Thrust Controller/6(rd)
  rd_d/1 -> Attitude Controleller/7(rd_d), Thrust Controller/7(rd_d)
  rd_dd/1 -> Attitude Controleller/8(rd_dd), Thrust Controller/8(rd_dd)
  Attitude Controleller/4(att_e) -> att_e/1
  rd_ddd/1 -> Attitude Controleller/9(rd_ddd), Thrust Controller/9(rd_ddd)
  rd_dddd/1 -> Attitude Controleller/10(rd_dddd), Thrust Controller/10(rd_dddd)
  int_e/1 -> Attitude Controleller/11(int_e), Thrust Controller/11(int_e)
  Thrust Controller/2(alt_e) -> alt_e/1
  Thrust Controller/1(F) -> F/1
  Attitude Controleller/3(torque_z) -> Terminator2/1
  euler angle/1 -> Yaw Controller/1(In1)
  Yaw Controller/1(torque_z) -> External Torque Observer/4(torque_z), torque_z/1
  External Torque Observer/1(omega_hat) -> Delay1/1
  Delay/1 -> Yaw Controller/2(ext torq), Attitude Controleller/12(ext_torq), External Torque Observer/5("ext_torque_hat ")
  External Torque Observer/2(ext_torque_hat) -> rd1/1, Delay/1  "rbt1 ext torq"
  Delay1/1 -> External Torque Observer/6("omega_hat ")
  time/1(real times) -> External Torque Observer/7(time)

== system controller13_AIS/Adaptive Controller 1/observer ==
  xyz : Inport
  euler : Inport  Port=2
  Rotaion : Subsystem
  lateral observer : Subsystem
  r : Outport
  r_dot : Outport  Port=2
  r_dotdot : Outport  Port=3
  R : Outport  Port=4
  Omega : Outport  Port=5
  Rdot : Outport  Port=6
  wires:
  lateral observer/1(r) -> r/1
  xyz/1 -> lateral observer/1(XYZ)
  lateral observer/2(r_dot) -> r_dot/1
  lateral observer/3(r_dotdot) -> r_dotdot/1
  Rotaion/1(R) -> R/1
  euler/1 -> Rotaion/1(Euler)
  Rotaion/2(Rdot) -> Rdot/1
  Rotaion/3(Omega) -> Omega/1

== system controller13_AIS/Adaptive Controller 1/time ==
  constant : Constant
  time : DiscreteIntegrator  gainval=1  SampleTime=-1  UpperSaturationLimit=1  LowerSaturationLimit=0  ICPrevOutput=DiscIntNeverNeededParam  ICPrevScaledInput=DiscIntNeverNeededParam
  real times : Outport
  wires:
  constant/1 -> time/1
  time/1 -> real times/1

== system controller13_AIS/Adaptive Controller 2/adaptive system ==
  att_e : Inport
  alt_e : Inport  Port=2
  Mux : Mux  Inputs=2
  Saturation1 : Saturate  UpperLimit=1  LowerLimit=-1
  Saturation3 : Saturate  UpperLimit=0.06  LowerLimit=-0.06
  Scope : Scope
  Unit Delay : UnitDelay  SampleTime=-1  HasFrameUpgradeWarning=on
  enable1 : Product  Inputs=**
  integral enable : Constant  Value=ctr2.integral.en
  integrator : Subsystem
  safety1 : Subsystem
  safety2 : Subsystem
  thrust offset : Constant  Value=flt.thrust_off
  torque offset : Constant  Value=[flt.torx_off;flt.tory_off;flt.torz_off]
  " tor_off" : Outport
  th_off : Outport  Port=2
  int_e : Outport  Port=3
  wires:
  torque offset/1 -> integrator/2(torque offset)
  thrust offset/1 -> integrator/3(thrust_offset)
  integrator/3(th_off) -> th_off/1
  integrator/1(int_e) -> Unit Delay/1
  integral enable/1 -> enable1/1
  Mux/1 -> integrator/1(e)
  Unit Delay/1 -> enable1/2
  integrator/2(" torq_off") -> Scope/1, " tor_off"/1
  att_e/1 -> safety1/1(In1)
  enable1/1 -> int_e/1
  alt_e/1 -> safety2/1(In1)
  Saturation1/1 -> Mux/1
  Saturation3/1 -> Mux/2
  safety1/1(Out1) -> Saturation1/1
  safety2/1(Out1) -> Saturation3/1

== system controller13_AIS/Adaptive Controller 2/attitude and thrust controller ==
  note: x_hat_pred
  r : Inport
  r_dot : Inport  Port=2
  r_dotdot : Inport  Port=3
  R : Inport  Port=4
  Omega : Inport  Port=5
  rd : Inport  Port=6
  rd_d : Inport  Port=7
  rd_dd : Inport  Port=8
  rd_ddd : Inport  Port=9
  rd_dddd : Inport  Port=10
  int_e : Inport  Port=11
  euler angle : Inport  Port=12
  Attitude Controleller : MATLAB Function  TreatAsAtomicUnit=on
  Delay : Delay  DelayLength=1  InitialCondition=ctr2.torque_obs.ext_torq_hat_init  SampleTime=mdl.T
  Delay1 : Delay  DelayLength=1  InitialCondition=ctr2.torque_obs.omega_hat_init  SampleTime=mdl.T
  External Torque Observer : MATLAB Function  TreatAsAtomicUnit=on
  Terminator2 : Terminator
  Thrust Controller : MATLAB Function  TreatAsAtomicUnit=on
  Yaw Controller : Subsystem
  rd1 : slrealtimeloglib/File Log  decimation=1
      settings: SourceProductBaseCode=XP
  time : Subsystem
  torque_x : Outport
  torque_y : Outport  Port=2
  torque_z : Outport  Port=3
  F : Outport  Port=4
  att_e : Outport  Port=5
  alt_e : Outport  Port=6
  wires:
  r/1 -> Thrust Controller/1(r), Attitude Controleller/1(r)
  Attitude Controleller/1(torque_x) -> External Torque Observer/2(torque_x), torque_x/1
  r_dot/1 -> Attitude Controleller/2(r_dot), Thrust Controller/2(r_dot)
  r_dotdot/1 -> Attitude Controleller/3(r_dotdot), Thrust Controller/3(r_dotdot)
  R/1 -> Attitude Controleller/4(R), Thrust Controller/4(R)
  Attitude Controleller/2(torque_y) -> External Torque Observer/3(torque_y), torque_y/1
  Omega/1 -> Attitude Controleller/5(Omega), External Torque Observer/1(omega), Thrust Controller/5(Omega)
  rd/1 -> Attitude Controleller/6(rd), Thrust Controller/6(rd)
  rd_d/1 -> Attitude Controleller/7(rd_d), Thrust Controller/7(rd_d)
  rd_dd/1 -> Attitude Controleller/8(rd_dd), Thrust Controller/8(rd_dd)
  Attitude Controleller/4(att_e) -> att_e/1
  rd_ddd/1 -> Attitude Controleller/9(rd_ddd), Thrust Controller/9(rd_ddd)
  rd_dddd/1 -> Attitude Controleller/10(rd_dddd), Thrust Controller/10(rd_dddd)
  int_e/1 -> Attitude Controleller/11(int_e), Thrust Controller/11(int_e)
  Thrust Controller/2(alt_e) -> alt_e/1
  Thrust Controller/1(F) -> F/1
  Attitude Controleller/3(torque_z) -> Terminator2/1
  euler angle/1 -> Yaw Controller/1(In1)
  Yaw Controller/1(torque_z) -> External Torque Observer/4(torque_z), torque_z/1
  External Torque Observer/1(omega_hat) -> Delay1/1
  Delay/1 -> Yaw Controller/2(ext torq), Attitude Controleller/12(ext_torq), External Torque Observer/5("ext_torque_hat ")
  External Torque Observer/2(ext_torque_hat) -> rd1/1, Delay/1  "rbt2 ext torq"
  Delay1/1 -> External Torque Observer/6("omega_hat ")
  time/1(real times) -> External Torque Observer/7(time)

== system controller13_AIS/Adaptive Controller 2/observer ==
  xyz : Inport
  euler : Inport  Port=2
  Rotaion : Subsystem
  lateral observer : Subsystem
  r : Outport
  r_dot : Outport  Port=2
  r_dotdot : Outport  Port=3
  R : Outport  Port=4
  Omega : Outport  Port=5
  Rdot : Outport  Port=6
  wires:
  lateral observer/1(r) -> r/1
  xyz/1 -> lateral observer/1(XYZ)
  lateral observer/2(r_dot) -> r_dot/1
  lateral observer/3(r_dotdot) -> r_dotdot/1
  Rotaion/1(R) -> R/1
  euler/1 -> Rotaion/1(Euler)
  Rotaion/2(Rdot) -> Rdot/1
  Rotaion/3(Omega) -> Omega/1

== system controller13_AIS/Adaptive Controller 2/observer1 ==
  xyz : Inport
  euler : Inport  Port=2
  f_cmd : Inport  Port=3
  tau_cmd_x : Inport  Port=4
  tau_cmd_y : Inport  Port=5
  Constant : Constant  Value=zeros(3,1)
  Constant1 : Constant  Value=zeros(9,1)
  Mux : Mux
  Overload Options : slrealtimetgmanagement/Overload Options  startupDur=100  startupDurSrc=Tunable Parameter  maxOverload=10  maxOverloadSrc=Tunable Parameter  TETFlag=on
      settings: SourceProductBaseCode=XP
  Terminator1 : Terminator  Commented=on
  Terminator2 : Terminator  Commented=on
  UKF : Subsystem  Commented=on
  UKF1 : Subsystem
  UKF2 : Subsystem  Commented=on
  eul to rotation matrix : MATLAB Function  TreatAsAtomicUnit=on
  lateral observer : Subsystem  Commented=on
  ukf_prediction_time : Constant  Value=ukf_prediction_time
  r : Outport
  r_dot : Outport  Port=2
  r_dotdot : Outport  Port=3
  R : Outport  Port=4
  Omega : Outport  Port=5
  Rdot : Outport  Port=6
  wires:
  euler/1 -> eul to rotation matrix/1(euler_angles)
  xyz/1 -> UKF1/1(r_in)
  UKF1/4(omega_out) -> Mux/4, Omega/1
  UKF1/3(R_out) -> R/1, Mux/3
  UKF1/2(r_dot_out) -> Mux/2, r_dot/1
  UKF1/1(r_out) -> Mux/1, r/1
  Constant1/1 -> Rdot/1
  Overload Options/2 -> Terminator1/1  "UKF TET"
  Overload Options/1 -> Terminator2/1  "UKF count"
  Mux/1 -> Overload Options/1
  ukf_prediction_time/1 -> UKF1/6(s_prediciton_time)
  Constant/1 -> r_dotdot/1
  eul to rotation matrix/1(R) -> UKF1/2(R_in)
  f_cmd/1 -> UKF1/3(f_cmd)
  tau_cmd_x/1 -> UKF1/4(tau_cmd_x)
  tau_cmd_y/1 -> UKF1/5(tau_cmd_y)

== system controller13_AIS/Adaptive Controller 2/time ==
  constant : Constant
  time : DiscreteIntegrator  gainval=1  SampleTime=-1  UpperSaturationLimit=1  LowerSaturationLimit=0  ICPrevOutput=DiscIntNeverNeededParam  ICPrevScaledInput=DiscIntNeverNeededParam
  real times : Outport
  wires:
  constant/1 -> time/1
  time/1 -> real times/1

== system controller13_AIS/Force//Torque to Trajectory Specs 1/force//torque to module thrust ==
  thrust : Inport
  x Tq : Inport  Port=2
  y Tq : Inport  Port=3
  z Tq : Inport  Port=4
  Mux : Mux
  SaturatingRamp : DiscreteIntegrator  gainval=1  SampleTime=-1  UpperSaturationLimit=1  LowerSaturationLimit=0  ICPrevOutput=DiscIntNeverNeededParam  ICPrevScaledInput=DiscIntNeverNeededParam
  constant : Constant
  mapping scheme (flipping compataible) : MATLAB Function  TreatAsAtomicUnit=on  SystemSampleTime=mdl.T
  module thrusts (1-4) : Outport  PortDimensions=4
  wires:
  thrust/1 -> Mux/1
  x Tq/1 -> Mux/2
  y Tq/1 -> Mux/3
  z Tq/1 -> Mux/4
  Mux/1 -> mapping scheme (flipping compataible)/2(inputs)
  mapping scheme (flipping compataible)/1(module_f) -> module thrusts (1-4)/1
  constant/1 -> SaturatingRamp/1
  SaturatingRamp/1 -> mapping scheme (flipping compataible)/1(time)

== system controller13_AIS/Force//Torque to Trajectory Specs 1/nominal desired voltage ==
  Force : Inport
  SaturatingRamp : DiscreteIntegrator  gainval=1  SampleTime=-1  UpperSaturationLimit=1  LowerSaturationLimit=0  ICPrevOutput=DiscIntNeverNeededParam  ICPrevScaledInput=DiscIntNeverNeededParam
  Switch : Switch  Criteria=u2 > Threshold
  constant1 : Constant
  "force to voltage (hovering) " : Subsystem
  force to voltage flipping : Subsystem
  map_selection : MATLAB Function  TreatAsAtomicUnit=on  SystemSampleTime=mdl.T
  Voltages : Outport
  wires:
  Force/1 -> force to voltage flipping/1(force), "force to voltage (hovering) "/1(force)
  "force to voltage (hovering) "/1(Vout) -> Switch/1
  force to voltage flipping/1(Vout) -> Switch/3
  Switch/1 -> Voltages/1
  map_selection/1(hover_map) -> Switch/2
  constant1/1 -> SaturatingRamp/1
  SaturatingRamp/1 -> map_selection/1(time)

== system controller13_AIS/Force//Torque to Trajectory Specs 2/force//torque to module thrust ==
  thrust : Inport
  x Tq : Inport  Port=2
  y Tq : Inport  Port=3
  z Tq : Inport  Port=4
  Mux : Mux
  SaturatingRamp : DiscreteIntegrator  gainval=1  SampleTime=-1  UpperSaturationLimit=1  LowerSaturationLimit=0  ICPrevOutput=DiscIntNeverNeededParam  ICPrevScaledInput=DiscIntNeverNeededParam
  constant : Constant
  mapping scheme (flipping compataible) : MATLAB Function  TreatAsAtomicUnit=on  SystemSampleTime=mdl.T
  module thrusts (1-4) : Outport  PortDimensions=4
  wires:
  thrust/1 -> Mux/1
  x Tq/1 -> Mux/2
  y Tq/1 -> Mux/3
  z Tq/1 -> Mux/4
  Mux/1 -> mapping scheme (flipping compataible)/2(inputs)
  mapping scheme (flipping compataible)/1(module_f) -> module thrusts (1-4)/1
  constant/1 -> SaturatingRamp/1
  SaturatingRamp/1 -> mapping scheme (flipping compataible)/1(time)

== system controller13_AIS/Force//Torque to Trajectory Specs 2/nominal desired voltage ==
  Force : Inport
  SaturatingRamp : DiscreteIntegrator  gainval=1  SampleTime=-1  UpperSaturationLimit=1  LowerSaturationLimit=0  ICPrevOutput=DiscIntNeverNeededParam  ICPrevScaledInput=DiscIntNeverNeededParam
  Switch : Switch  Criteria=u2 > Threshold
  constant1 : Constant
  "force to voltage (hovering) " : Subsystem
  force to voltage flipping : Subsystem
  map_selection : MATLAB Function  TreatAsAtomicUnit=on  SystemSampleTime=mdl.T
  Voltages : Outport
  wires:
  Force/1 -> force to voltage flipping/1(force), "force to voltage (hovering) "/1(force)
  "force to voltage (hovering) "/1(Vout) -> Switch/1
  force to voltage flipping/1(Vout) -> Switch/3
  Switch/1 -> Voltages/1
  map_selection/1(hover_map) -> Switch/2
  constant1/1 -> SaturatingRamp/1
  SaturatingRamp/1 -> map_selection/1(time)

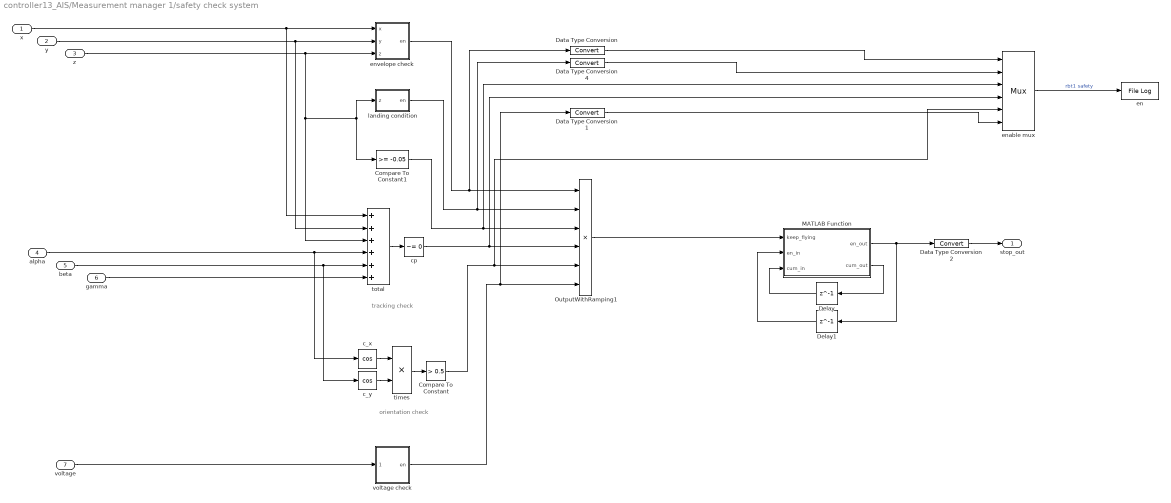
== system controller13_AIS/Measurement manager 1/safety check system ==
  note: orientation check
  note: tracking check
  x : Inport
  y : Inport  Port=2
  z : Inport  Port=3
  alpha : Inport  Port=4
  beta : Inport  Port=5
  gamma : Inport  Port=6
  voltage : Inport  Port=7
  Compare To Constant : simulink/Logic and Bit Operations/Compare To Constant  relop=>  const=0.5  OutDataTypeStr=uint8
  Compare To Constant1 : simulink/Logic and Bit Operations/Compare To Constant  relop=>=  const=-0.05  OutDataTypeStr=uint8
  Data Type Conversion{,1..2,4} (4 alike) : DataTypeConversion
  Delay : Delay  DelayLength=1
  Delay1 : Delay  DelayLength=1  InitialCondition=1
  MATLAB Function : MATLAB Function  TreatAsAtomicUnit=on
  OutputWithRamping1 : Product  Inputs=6  RndMeth=Zero
  c_x : Trigonometry  Operator=cos
  c_y : Trigonometry  Operator=cos
  cp : simulink/Logic and Bit Operations/Compare To Zero  relop=~=  OutDataTypeStr=uint8
  en : slrealtimeloglib/File Log  decimation=1
      settings: SourceProductBaseCode=XP
  enable mux : Mux  Inputs=6
      settings: DisplayOption=signals
  envelope check : MATLAB Function  TreatAsAtomicUnit=on
  landing condition : Subsystem
  times : Product  RndMeth=Zero
  total : Sum  Inputs=++++++
  voltage check : MATLAB Function  TreatAsAtomicUnit=on  SystemSampleTime=mdl.T
  stop_out : Outport
  wires:
  Compare To Constant1/1 -> enable mux/3, OutputWithRamping1/3
  y/1 -> envelope check/2(y), total/2
  cp/1 -> enable mux/4, OutputWithRamping1/4
  envelope check/1(en) -> Data Type Conversion/1, OutputWithRamping1/1
  enable mux/1 -> en/1  "rbt1 safety"
  landing condition/1(en) -> Data Type Conversion4/1, OutputWithRamping1/2
  Data Type Conversion/1 -> enable mux/1
  times/1 -> Compare To Constant/1
  voltage check/1(en) -> Data Type Conversion1/1, OutputWithRamping1/6
  z/1 -> total/3, Compare To Constant1/1, landing condition/1(z), envelope check/3(z)
  Compare To Constant/1 -> enable mux/5, OutputWithRamping1/5
  total/1 -> cp/1
  Data Type Conversion4/1 -> enable mux/2
  x/1 -> total/1, envelope check/1(x)
  alpha/1 -> total/4, c_x/1
  beta/1 -> total/5, c_y/1
  c_x/1 -> times/1
  c_y/1 -> times/2
  Data Type Conversion1/1 -> enable mux/6
  voltage/1 -> voltage check/1(voltage)
  gamma/1 -> total/6
  OutputWithRamping1/1 -> MATLAB Function/1(keep_flying)
  Delay1/1 -> MATLAB Function/2(en_in)
  MATLAB Function/1(en_out) -> Delay1/1, Data Type Conversion2/1
  Delay/1 -> MATLAB Function/3(cum_in)
  MATLAB Function/2(cum_out) -> Delay/1
  Data Type Conversion2/1 -> stop_out/1

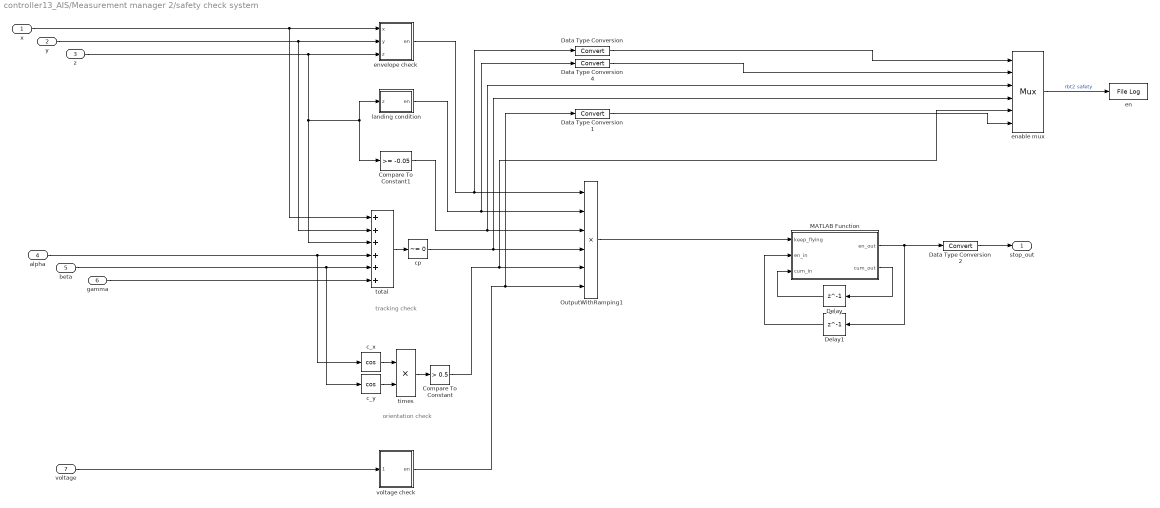
== system controller13_AIS/Measurement manager 2/safety check system ==
  note: orientation check
  note: tracking check
  x : Inport
  y : Inport  Port=2
  z : Inport  Port=3
  alpha : Inport  Port=4
  beta : Inport  Port=5
  gamma : Inport  Port=6
  voltage : Inport  Port=7
  Compare To Constant : simulink/Logic and Bit Operations/Compare To Constant  relop=>  const=0.5  OutDataTypeStr=uint8
  Compare To Constant1 : simulink/Logic and Bit Operations/Compare To Constant  relop=>=  const=-0.05  OutDataTypeStr=uint8
  Data Type Conversion{,1..2,4} (4 alike) : DataTypeConversion
  Delay : Delay  DelayLength=1
  Delay1 : Delay  DelayLength=1  InitialCondition=1
  MATLAB Function : MATLAB Function  TreatAsAtomicUnit=on
  OutputWithRamping1 : Product  Inputs=6  RndMeth=Zero
  c_x : Trigonometry  Operator=cos
  c_y : Trigonometry  Operator=cos
  cp : simulink/Logic and Bit Operations/Compare To Zero  relop=~=  OutDataTypeStr=uint8
  en : slrealtimeloglib/File Log  decimation=1
      settings: SourceProductBaseCode=XP
  enable mux : Mux  Inputs=6
      settings: DisplayOption=signals
  envelope check : MATLAB Function  TreatAsAtomicUnit=on
  landing condition : Subsystem
  times : Product  RndMeth=Zero
  total : Sum  Inputs=++++++
  voltage check : MATLAB Function  TreatAsAtomicUnit=on  SystemSampleTime=mdl.T
  stop_out : Outport
  wires:
  Compare To Constant1/1 -> enable mux/3, OutputWithRamping1/3
  y/1 -> envelope check/2(y), total/2
  cp/1 -> enable mux/4, OutputWithRamping1/4
  envelope check/1(en) -> Data Type Conversion/1, OutputWithRamping1/1
  enable mux/1 -> en/1  "rbt2 safety"
  landing condition/1(en) -> Data Type Conversion4/1, OutputWithRamping1/2
  Data Type Conversion/1 -> enable mux/1
  times/1 -> Compare To Constant/1
  voltage check/1(en) -> Data Type Conversion1/1, OutputWithRamping1/6
  z/1 -> total/3, Compare To Constant1/1, landing condition/1(z), envelope check/3(z)
  Compare To Constant/1 -> enable mux/5, OutputWithRamping1/5
  total/1 -> cp/1
  Data Type Conversion4/1 -> enable mux/2
  x/1 -> total/1, envelope check/1(x)
  alpha/1 -> total/4, c_x/1
  beta/1 -> total/5, c_y/1
  c_x/1 -> times/1
  c_y/1 -> times/2
  Data Type Conversion1/1 -> enable mux/6
  voltage/1 -> voltage check/1(voltage)
  gamma/1 -> total/6
  OutputWithRamping1/1 -> MATLAB Function/1(keep_flying)
  Delay1/1 -> MATLAB Function/2(en_in)
  MATLAB Function/1(en_out) -> Delay1/1, Data Type Conversion2/1
  Delay/1 -> MATLAB Function/3(cum_in)
  MATLAB Function/2(cum_out) -> Delay/1
  Data Type Conversion2/1 -> stop_out/1

== system controller13_AIS/Phantom trigger/timer1 ==
  SaturatingRamp : DiscreteIntegrator  gainval=1  SampleTime=-1  UpperSaturationLimit=1  LowerSaturationLimit=0  ICPrevOutput=DiscIntNeverNeededParam  ICPrevScaledInput=DiscIntNeverNeededParam
  constant : Constant
  time : Outport
  wires:
  constant/1 -> SaturatingRamp/1
  SaturatingRamp/1 -> time/1
